simulink model "simulas1"  (R2023a)
settings: Solver=VariableStepAuto  StartTime=0.0  StopTime=10.0  RelTol=1e-3
libraries: simulink x4
settings Model: Creator=a2408732  LastModifiedBy=a2408732

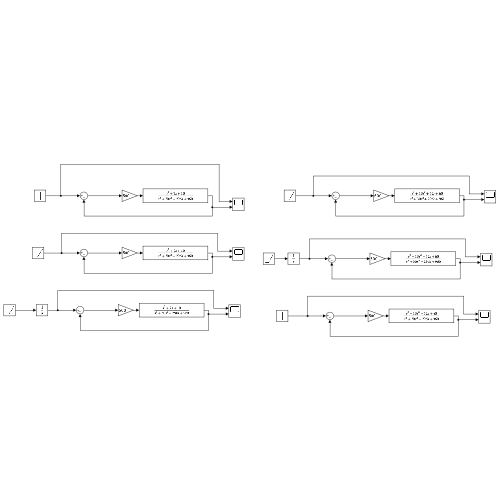
[thumbnail: Simulink's stored preview of the top-level diagram]
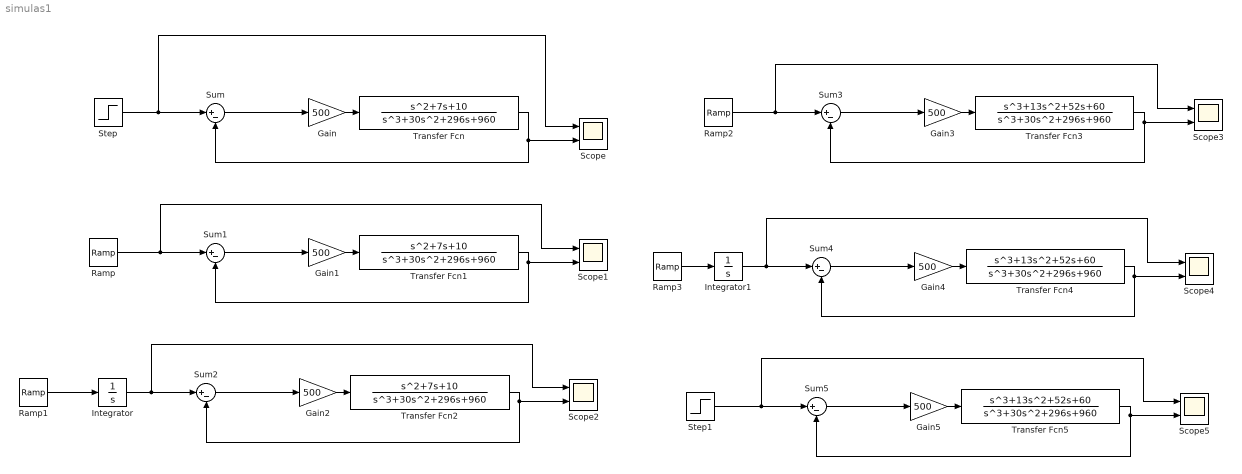
== system simulas1 ==
  Gain{,1..5} (6 alike) : Gain  Gain=500
  Integrator : Integrator
  Integrator1 : Integrator
  Ramp{,1..3} (4 alike) : simulink/Sources/Ramp  slope=1  start=0  InitialOutput=0
  Scope{,1..5} (6 alike) : Scope  NumInputPorts=2
  Step : Step  SampleTime=0
  Step1 : Step  SampleTime=0
  Sum{,1..5} (6 alike) : Sum  Inputs=|+-
  Transfer Fcn : TransferFcn  Numerator=[1 7 10]  Denominator=[1 30 296 960]
  Transfer Fcn1 : TransferFcn  Numerator=[1 7 10]  Denominator=[1 30 296 960]
  Transfer Fcn2 : TransferFcn  Numerator=[1 7 10]  Denominator=[1 30 296 960]
  Transfer Fcn3 : TransferFcn  Numerator=[1 13 52 60]  Denominator=[1 30 296 960]
  Transfer Fcn4 : TransferFcn  Numerator=[1 13 52 60]  Denominator=[1 30 296 960]
  Transfer Fcn5 : TransferFcn  Numerator=[1 13 52 60]  Denominator=[1 30 296 960]
  wires:
  Sum/1 -> Gain/1
  Gain/1 -> Transfer Fcn/1
  Transfer Fcn/1 -> Sum/2, Scope/2
  Transfer Fcn1/1 -> Sum1/2, Scope1/2
  Gain1/1 -> Transfer Fcn1/1
  Sum1/1 -> Gain1/1
  Step/1 -> Scope/1, Sum/1
  Ramp/1 -> Scope1/1, Sum1/1
  Sum2/1 -> Gain2/1
  Gain2/1 -> Transfer Fcn2/1
  Transfer Fcn2/1 -> Sum2/2, Scope2/2
  Ramp1/1 -> Integrator/1
  Integrator/1 -> Scope2/1, Sum2/1
  Sum3/1 -> Gain3/1
  Gain3/1 -> Transfer Fcn3/1
  Transfer Fcn3/1 -> Sum3/2, Scope3/2
  Ramp2/1 -> Scope3/1, Sum3/1
  Transfer Fcn4/1 -> Sum4/2, Scope4/2
  Gain4/1 -> Transfer Fcn4/1
  Ramp3/1 -> Integrator1/1
  Sum4/1 -> Gain4/1
  Integrator1/1 -> Scope4/1, Sum4/1
  Transfer Fcn5/1 -> Sum5/2, Scope5/2
  Gain5/1 -> Transfer Fcn5/1
  Step1/1 -> Scope5/1, Sum5/1
  Sum5/1 -> Gain5/1
